simulink subsystem "weHaveExecutiveControllerAtHome"  (R2025b)
settings: Solver=VariableStepAuto  StartTime=0.0  StopTime=10.0  RelTol=1e-3
settings Model: Creator=koryh  LastModifiedBy=kjhaydon

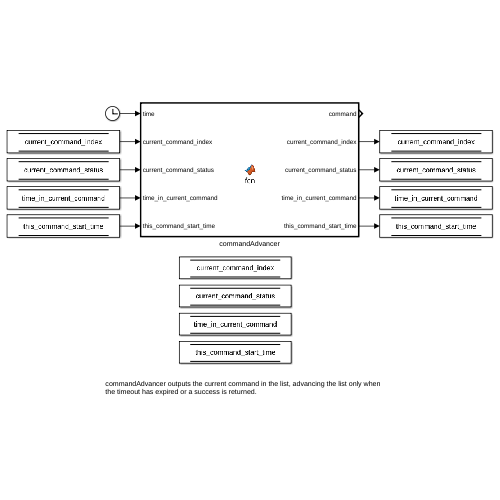
[thumbnail: Simulink's stored preview of the top-level diagram]
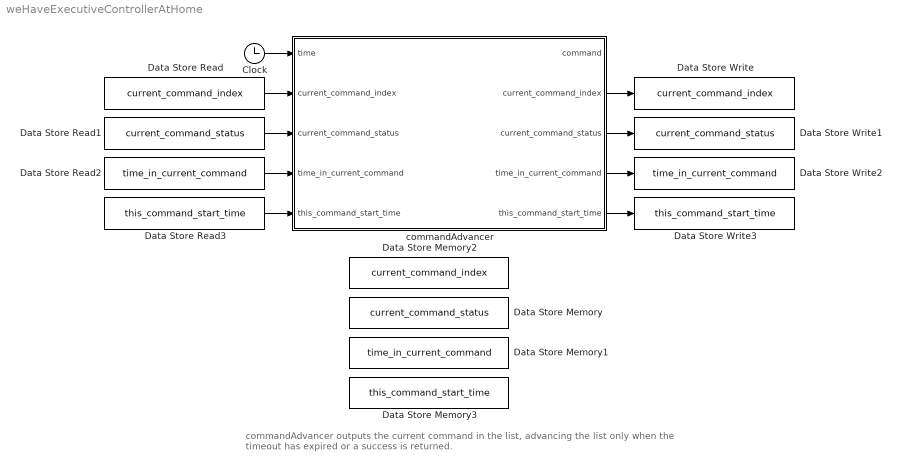
== system weHaveExecutiveControllerAtHome ==
  note: commandAdvancer outputs the current command in the list, advancing the list only when the timeout has expired or a success is returned.
  Clock : Clock
  Data Store Memory : DataStoreMemory  DataStoreName=current_command_status  WriteAfterWriteMsg=warning  InitialValue=uint8('SUCC')  ShowAdditionalParam=off  OutDataTypeStr=uint8
  Data Store Memory1 : DataStoreMemory  DataStoreName=time_in_current_command  WriteAfterWriteMsg=warning  ShowAdditionalParam=off  OutDataTypeStr=uint8
  Data Store Memory2 : DataStoreMemory  DataStoreName=current_command_index  WriteAfterWriteMsg=warning  ShowAdditionalParam=off  OutDataTypeStr=uint8
  Data Store Memory3 : DataStoreMemory  DataStoreName=this_command_start_time  WriteAfterWriteMsg=warning  ShowAdditionalParam=off  OutDataTypeStr=uint8
  Data Store Read : DataStoreRead  DataStoreName=current_command_index  IndexOptions=Index vector (dialog)  Indices=1  OutputSizes=1
  Data Store Read1 : DataStoreRead  DataStoreName=current_command_status  IndexOptions=Index vector (dialog)  Indices=1  OutputSizes=1
  Data Store Read2 : DataStoreRead  DataStoreName=time_in_current_command  IndexOptions=Index vector (dialog)  Indices=1  OutputSizes=1
  Data Store Read3 : DataStoreRead  DataStoreName=this_command_start_time  IndexOptions=Index vector (dialog)  Indices=1  OutputSizes=1
  Data Store Write : DataStoreWrite  DataStoreName=current_command_index  IndexOptions=Index vector (dialog)  Indices=1  OutputSizes=1
  Data Store Write1 : DataStoreWrite  DataStoreName=current_command_status  IndexOptions=Index vector (dialog)  Indices=1  OutputSizes=1
  Data Store Write2 : DataStoreWrite  DataStoreName=time_in_current_command  IndexOptions=Index vector (dialog)  Indices=1  OutputSizes=1
  Data Store Write3 : DataStoreWrite  DataStoreName=this_command_start_time  IndexOptions=Index vector (dialog)  Indices=1  OutputSizes=1
  commandAdvancer : MATLAB Function  TreatAsAtomicUnit=on
  wires:
  Clock/1 -> commandAdvancer/1(time)
  Data Store Read/1 -> commandAdvancer/2("current_command_index ")
  Data Store Read1/1 -> commandAdvancer/3("current_command_status ")
  commandAdvancer/2(current_command_index) -> Data Store Write/1
  Data Store Read2/1 -> commandAdvancer/4("time_in_current_command ")
  commandAdvancer/3(current_command_status) -> Data Store Write1/1
  commandAdvancer/4(time_in_current_command) -> Data Store Write2/1
  commandAdvancer/5(this_command_start_time) -> Data Store Write3/1
  Data Store Read3/1 -> commandAdvancer/5("this_command_start_time ")

== matlab function weHaveExecutiveControllerAtHome/commandAdvancer ==
  data: time input; command output; mission parameter; current_command_index input; current_command_index output; current_command_status input; current_command_status output; time_in_current_command input; time_in_current_command output; this_command_start_time input; this_command_start_time output
function [command, current_command_index, current_command_status, time_in_current_command, this_command_start_time] = fcn(time, mission, current_command_index, current_command_status, time_in_current_command, this_command_start_time)

[command, current_command_index, current_command_status, time_in_current_command, this_command_start_time] = commandAdvancer(time, mission, current_command_index, current_command_status, time_in_current_command, this_command_start_time);
